simulink model "model1"  (R2022a)
settings: Solver=VariableStepAuto  StartTime=0.0  StopTime=0.2  MaxStep=1e-4  RelTol=1e-3
values from neighbouring files (symbols this model uses):
  C12 = 444    [config.m]
  J1 = 0.0077    [config.m]
  J2 = 0.0023    [config.m]
  M1 = 0.1*Mnom    [task1.m]
settings Model: Creator=Vvlad  LastModifiedBy=Vvlad

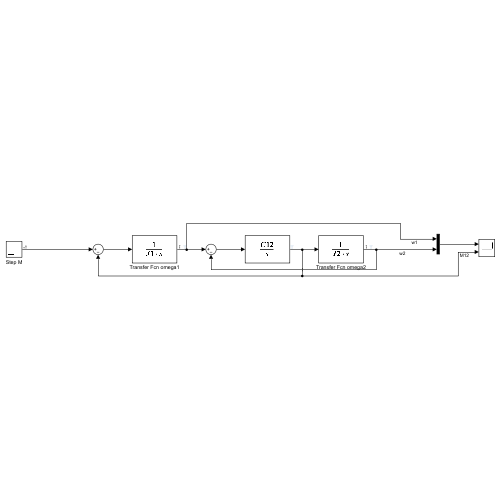
[thumbnail: Simulink's stored preview of the top-level diagram]
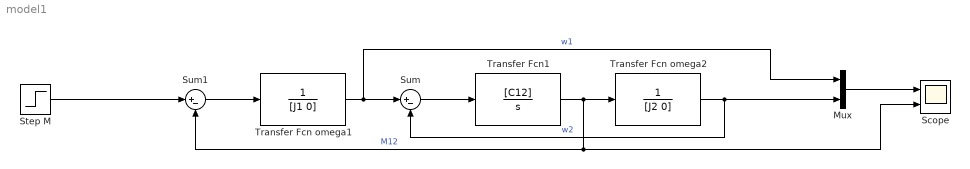
== system model1 ==
  Mux : Mux  Inputs=2
  Scope : Scope  NumInputPorts=2
  Step M : Step  Time=0  After=M1  SampleTime=0
  Sum : Sum  Inputs=|+-
  Sum1 : Sum  Inputs=|+-
  Transfer Fcn omega1 : TransferFcn  Denominator=[J1 0]
  Transfer Fcn omega2 : TransferFcn  Denominator=[J2 0]
  Transfer Fcn1 : TransferFcn  Numerator=[C12]  Denominator=[1 0]
  wires:
  Sum/1 -> Transfer Fcn1/1
  Transfer Fcn omega1/1 -> Mux/1, Sum/1  "w1"
  Transfer Fcn1/1 -> Sum1/2, Scope/2, Transfer Fcn omega2/1  "M12"
  Sum1/1 -> Transfer Fcn omega1/1
  Mux/1 -> Scope/1
  Transfer Fcn omega2/1 -> Mux/2, Sum/2  "w2"
  Step M/1 -> Sum1/1
